simulink model "richvspoor"  (R2020b)
settings: Solver=VariableStepAuto  StartTime=0.0  StopTime=10.0  RelTol=1e-3
values from neighbouring files (symbols this model uses):
  i = 0.05    [main.m]
  r = 0.1    [main.m]
  sigma = 1    [main.m]
  Td = 0    [main.m]
  Tk = 2    [main.m]
  Tw = 0.1    [main.m]
libraries: dspsrcs4 x1
settings Model: Creator=erlended  LastModifiedBy=erlenddahlen

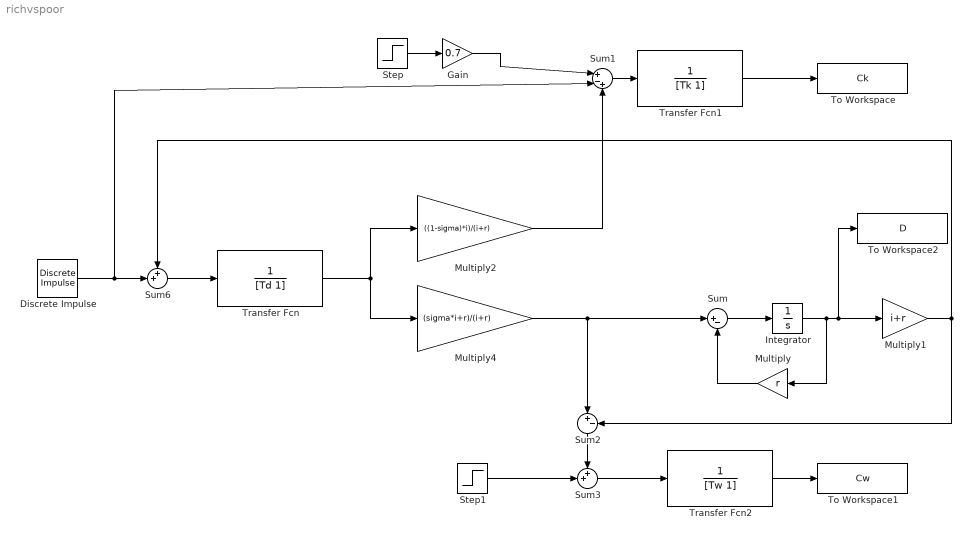
== system richvspoor ==
  Discrete Impulse : dspsrcs4/Discrete  Impulse  Delay=30  SampleTime=1  FrameSample=1  OutputFrames=off  dataType=double  isSigned=on  wordLen=16  udDataType=sfix(16)  fracBitsMode=Best precision  numFracBits=15  OutDataTypeStr=double  LastOutDataTypeStr=double
  Gain : Gain  Gain=0.7
  Integrator : Integrator
  Multiply : Gain  Gain=r
  Multiply1 : Gain  Gain=i+r
  Multiply2 : Gain  Gain=((1-sigma)*i)/(i+r)
  Multiply4 : Gain  Gain=(sigma*i+r)/(i+r)
  Step : Step  SampleTime=0
  Step1 : Step  SampleTime=0
  Sum : Sum  Inputs=|+-
  Sum1 : Sum  Inputs=|+-+
  Sum2 : Sum  Inputs=|+-
  Sum3 : Sum  Inputs=++|
  Sum6 : Sum  Inputs=++|
  To Workspace : ToWorkspace  VariableName=Ck  SaveFormat=Timeseries  SampleTime=-1
  To Workspace1 : ToWorkspace  VariableName=Cw  SaveFormat=Timeseries  SampleTime=-1
  To Workspace2 : ToWorkspace  VariableName=D  SaveFormat=Timeseries  SampleTime=-1
  Transfer Fcn : TransferFcn  Denominator=[Td 1]
  Transfer Fcn1 : TransferFcn  Denominator=[Tk 1]
  Transfer Fcn2 : TransferFcn  Denominator=[Tw 1]
  wires:
  Sum/1 -> Integrator/1
  Integrator/1 -> To Workspace2/1, Multiply1/1, Multiply/1
  Multiply/1 -> Sum/2
  Multiply1/1 -> Sum6/1, Sum2/2
  Sum1/1 -> Transfer Fcn1/1
  Step/1 -> Gain/1
  Transfer Fcn1/1 -> To Workspace/1
  Transfer Fcn/1 -> Multiply4/1, Multiply2/1
  Multiply2/1 -> Sum1/3
  Multiply4/1 -> Sum2/1, Sum/1
  Sum2/1 -> Sum3/1
  Step1/1 -> Sum3/2
  Sum3/1 -> Transfer Fcn2/1
  Transfer Fcn2/1 -> To Workspace1/1
  Sum6/1 -> Transfer Fcn/1
  Discrete Impulse/1 -> Sum6/2, Sum1/2
  Gain/1 -> Sum1/1
